simulink model "distortion"  (R2024a)
settings: Solver=VariableStepAuto  StartTime=0.0  StopTime=120  RelTol=1e-3
libraries: dspsnks4 x1, dspvision x1
settings Model: Creator=EAGLEAORUS  LastModifiedBy=fermata

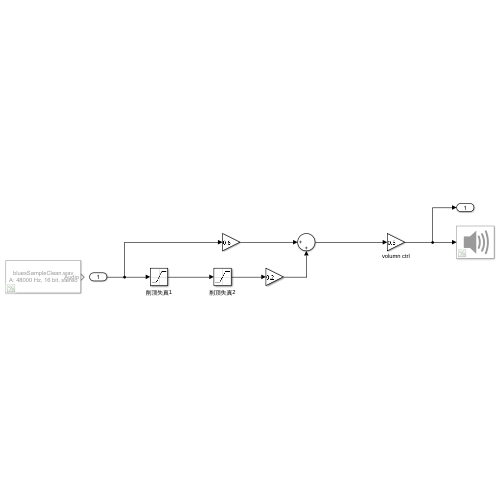
[thumbnail: Simulink's stored preview of the top-level diagram]
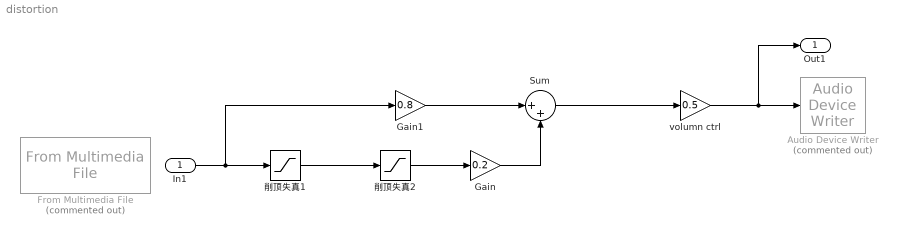
== system distortion ==
  In1 : Inport  OutDataTypeStr=int32
  Audio Device Writer : dspsnks4/Audio Device Writer  Commented=on  Driver=ALSA  Device=Default  InheritSampleRate=on  SampleRate=44100  BitDepth=16-bit integer  BufferSize=4096  NumBuffers=10  DefaultOutputChannelMapping=on  OutputChannelMapping=1:2  OutputNumUnderrunSamples=off  DriverIdx=8  DeviceWarnFlag=''
  From Multimedia File : dspvision/From Multimedia File  Commented=on  inputFilename=/home/fermata/Development/FPGA/patatodsp/doc/ADSD/Code/examples/simulink-common/bluesSampleClean.wav  readRange=[1 Inf]  loop=on  numPlays=inf  outputStreams=Audio only  videoDataType=single  audioDataType=int16  inheritSampleTime=on  userDefinedSampleTime=1/30  noAudioOutput=off  isIntensityVideo=off  fourcc=RGB  colorVideoFormat=Separate color signals  outputEOF=off  dataOrg=Column-major  audioFrameSize=1024  computeAudioFrameSize=off  outSamplingMode=Sample based
      settings: LibrarySourceBlock=audiosources/From Multimedia File
  Gain : Gain  Gain=0.2
  Gain1 : Gain  Gain=0.8
  Sum : Sum  Inputs=|++
  volumn ctrl : Gain  Gain=0.5  OutDataTypeStr=int32  SaturateOnIntegerOverflow=on
  削顶失真1 : Saturate  UpperLimit=0.2  LowerLimit=-0.2
  削顶失真2 : Saturate  UpperLimit=0.1  LowerLimit=-0.1  RndMeth=Convergent
  Out1 : Outport  OutDataTypeStr=int32  VectorParamsAs1DForOutWhenUnconnected=off
  wires:
  削顶失真1/1 -> 削顶失真2/1
  削顶失真2/1 -> Gain/1
  Sum/1 -> volumn ctrl/1
  volumn ctrl/1 -> Out1/1, Audio Device Writer/1
  Gain/1 -> Sum/2
  Gain1/1 -> Sum/1
  In1/1 -> Gain1/1, 削顶失真1/1
